simulink model "sim_test_sfunc"  (R2015a)
settings: Solver=ode45  StartTime=0.0  StopTime=10  MaxStep=0.1  RelTol=1e-3
settings Model: Creator=ut  LastModifiedBy=sj
settings DataIOCC: SignalLoggingSaveFormat=ModelDataLogs
settings OptimizationCC: ExpressionDepthLimit=2147483647  InitFltsAndDblsToZero=on
settings DebuggingCC: SaveWithParameterizedLinksMsg=none  UnderspecifiedInitializationDetection=Classic  MergeDetectMultiDrivingBlocksExec=none  SignalResolutionControl=TryResolveAllWithWarning  SolverPrmCheckMsg=warning  MultiTaskDSMMsg=warning  MultiTaskCondExecSysMsg=none  FcnCallInpInsideContextMsg=UseLocalSettings  StateNameClashWarn=warning
settings GRTTargetCC: TargetFcnLib=ansi_tfl_tmw.mat  CombineOutputUpdateFcns=off  GRTInterface=on

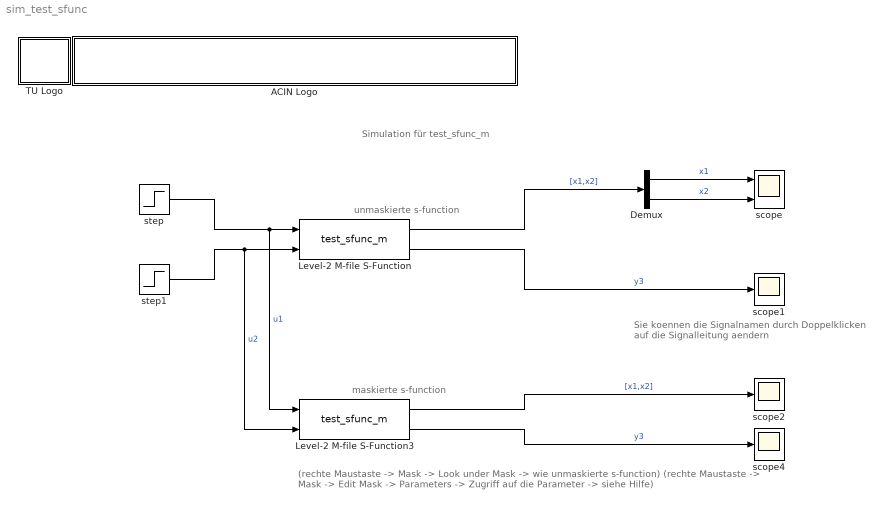
== system sim_test_sfunc ==
  note: Simulation für test_sfunc_m
  note: unmaskierte s-function
  note: maskierte s-function
  note: (rechte Maustaste -> Mask -> Look under Mask -> wie unmaskierte s-function)
      | (rechte Maustaste -> Mask -> Edit Mask -> Parameters -> Zugriff auf die Parameter -> siehe Hilfe)
  note: Sie koennen die Signalnamen durch
      | Doppelklicken auf die Signalleitung aendern
  ACIN Logo : Subsystem
      mask init:
      | s = get_param(gcb,'UserData');
      mask Display:
      | image(s.logo,[0 0 439 45]);
      | %axis image
  Demux : Demux  Outputs=2
  Level-2 M-file S-Function : M-S-Function  FunctionName=test_sfunc_m  Parameters=1,1,[0,1]
  Level-2 M-file S-Function3 : M-S-Function  FunctionName=test_sfunc_m  Parameters=a,b,x0  mask{a=1, b=1, x0=[0,1]}
      mask prompts: a "Parameter a"; b "Parameter b"; x0 "Anfangszustand x0"
      mask Display: disp('masked test_sfunc_m')
  TU Logo : Subsystem
      mask init:
      | s = get_param(gcb,'UserData');
      mask Display: image(s.logo,[0 0 45 45]);
  scope : Scope  NumInputPorts=2
      settings: YMin=-5~-5  YMax=5~5
  scope1 : Scope
  scope2 : Scope
      settings: SaveName=ScopeData3
  scope4 : Scope
      settings: SaveName=ScopeData2
  step : Step  After=0  SampleTime=0
  step1 : Step  Time=2  After=0  SampleTime=0
  wires:
  step/1 -> Level-2 M-file S-Function/1, Level-2 M-file S-Function3/1  "u1"
  step1/1 -> Level-2 M-file S-Function/2, Level-2 M-file S-Function3/2  "u2"
  Level-2 M-file S-Function/2 -> scope1/1  "y3"
  Level-2 M-file S-Function3/1 -> scope2/1  "[x1,x2]"
  Level-2 M-file S-Function3/2 -> scope4/1  "y3"
  Demux/1 -> scope/1  "x1"
  Demux/2 -> scope/2  "x2"
  Level-2 M-file S-Function/1 -> Demux/1  "[x1,x2]"

== system sim_test_sfunc/ACIN Logo ==

== system sim_test_sfunc/TU Logo ==
